simulink model "SAR_sw_neg"  (R2018b)
settings: Solver=VariableStepAuto  StartTime=0.0  StopTime=10.0  RelTol=1e-3
libraries: simulink_extras x11
settings Model: Creator=iamcy  LastModifiedBy=iamcy

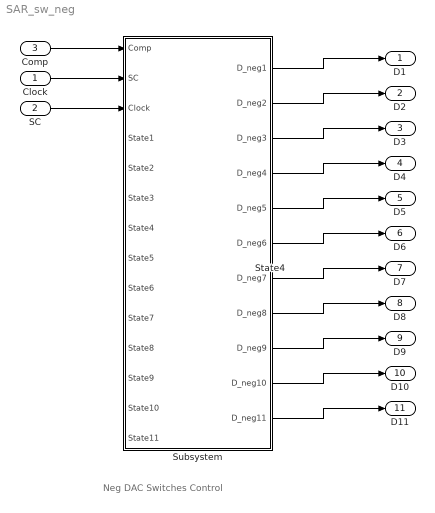
== system SAR_sw_neg ==
  note: Neg DAC Switches Control
  Clock : Inport
  SC : Inport  Port=2
  Comp : Inport  Port=3
  State4 : Inport  Port=4
  Subsystem : Subsystem
  D1 : Outport
  D2 : Outport  Port=2
  D3 : Outport  Port=3
  D4 : Outport  Port=4
  D5 : Outport  Port=5
  D6 : Outport  Port=6
  D7 : Outport  Port=7
  D8 : Outport  Port=8
  D9 : Outport  Port=9
  D10 : Outport  Port=10
  D11 : Outport  Port=11
  wires:
  Comp/1 -> Subsystem/1(Comp)
  Clock/1 -> Subsystem/2(SC)
  SC/1 -> Subsystem/3(Clock)
  Subsystem/1(D_neg1) -> D1/1
  Subsystem/2(D_neg2) -> D2/1
  Subsystem/3(D_neg3) -> D3/1
  Subsystem/4(D_neg4) -> D4/1
  Subsystem/5(D_neg5) -> D5/1
  Subsystem/6(D_neg6) -> D6/1
  Subsystem/7(D_neg7) -> D7/1
  Subsystem/8(D_neg8) -> D8/1
  Subsystem/9(D_neg9) -> D9/1
  Subsystem/10(D_neg10) -> D10/1
  Subsystem/11(D_neg11) -> D11/1

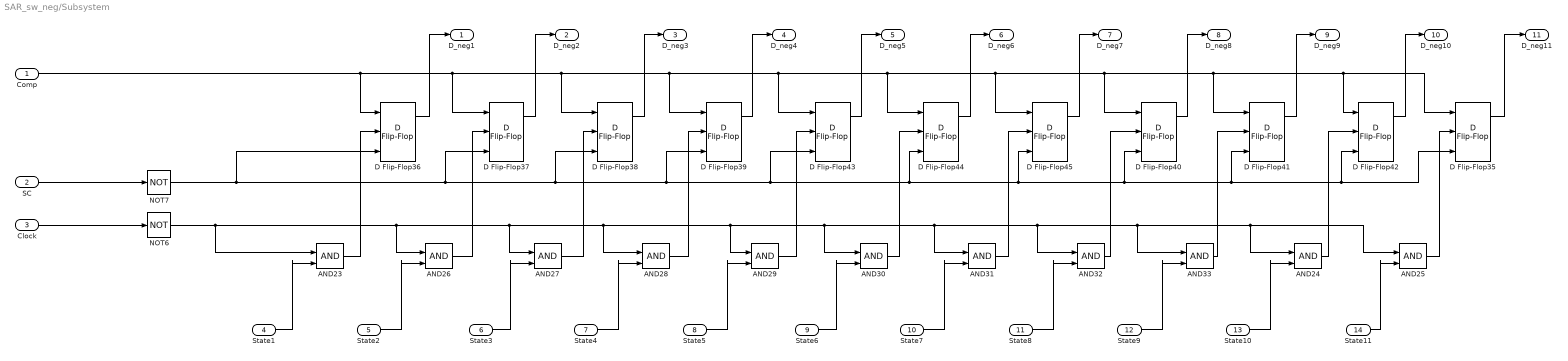
== system SAR_sw_neg/Subsystem ==
  Comp : Inport
  SC : Inport  Port=2
  Clock : Inport  Port=3
  State1 : Inport  Port=4
  State2 : Inport  Port=5
  State3 : Inport  Port=6
  State4 : Inport  Port=7
  State5 : Inport  Port=8
  State6 : Inport  Port=9
  State7 : Inport  Port=10
  State8 : Inport  Port=11
  State9 : Inport  Port=12
  State10 : Inport  Port=13
  State11 : Inport  Port=14
  AND{23..33} (11 alike) : Logic  IconShape=distinctive  AllPortsSameDT=off  OutDataTypeStr=boolean
  D Flip-Flop{35..45} (11 alike) : simulink_extras/Flip Flops/D Flip-Flop
      settings: SourceProductName=Simulink
  NOT6 : Logic  Operator=NOT  IconShape=distinctive  AllPortsSameDT=off  OutDataTypeStr=boolean
  NOT7 : Logic  Operator=NOT  IconShape=distinctive  AllPortsSameDT=off  OutDataTypeStr=boolean
  D_neg1 : Outport
  D_neg2 : Outport  Port=2
  D_neg3 : Outport  Port=3
  D_neg4 : Outport  Port=4
  D_neg5 : Outport  Port=5
  D_neg6 : Outport  Port=6
  D_neg7 : Outport  Port=7
  D_neg8 : Outport  Port=8
  D_neg9 : Outport  Port=9
  D_neg10 : Outport  Port=10
  D_neg11 : Outport  Port=11
  wires:
  NOT7/1 -> D Flip-Flop35/3, D Flip-Flop42/3, D Flip-Flop41/3, D Flip-Flop40/3, D Flip-Flop45/3, D Flip-Flop44/3, D Flip-Flop43/3, D Flip-Flop39/3, D Flip-Flop38/3, D Flip-Flop37/3, D Flip-Flop36/3
  D Flip-Flop41/1 -> D_neg9/1
  AND23/1 -> D Flip-Flop36/2
  State9/1 -> AND33/2
  Comp/1 -> D Flip-Flop35/1, D Flip-Flop42/1, D Flip-Flop41/1, D Flip-Flop40/1, D Flip-Flop45/1, D Flip-Flop44/1, D Flip-Flop43/1, D Flip-Flop39/1, D Flip-Flop38/1, D Flip-Flop37/1, D Flip-Flop36/1
  D Flip-Flop42/1 -> D_neg10/1
  AND27/1 -> D Flip-Flop38/2
  NOT6/1 -> AND25/1, AND24/1, AND33/1, AND32/1, AND31/1, AND30/1, AND29/1, AND28/1, AND27/1, AND26/1, AND23/1
  AND25/1 -> D Flip-Flop35/2
  AND29/1 -> D Flip-Flop43/2
  AND31/1 -> D Flip-Flop45/2
  AND28/1 -> D Flip-Flop39/2
  State1/1 -> AND23/2
  AND33/1 -> D Flip-Flop41/2
  D Flip-Flop45/1 -> D_neg7/1
  State5/1 -> AND29/2
  AND26/1 -> D Flip-Flop37/2
  AND24/1 -> D Flip-Flop42/2
  SC/1 -> NOT7/1
  AND32/1 -> D Flip-Flop40/2
  State10/1 -> AND24/2
  AND30/1 -> D Flip-Flop44/2
  D Flip-Flop38/1 -> D_neg3/1
  Clock/1 -> NOT6/1
  D Flip-Flop36/1 -> D_neg1/1
  D Flip-Flop37/1 -> D_neg2/1
  D Flip-Flop35/1 -> D_neg11/1
  D Flip-Flop43/1 -> D_neg5/1
  State4/1 -> AND28/2
  State3/1 -> AND27/2
  State2/1 -> AND26/2
  State8/1 -> AND32/2
  D Flip-Flop44/1 -> D_neg6/1
  State6/1 -> AND30/2
  State11/1 -> AND25/2
  D Flip-Flop40/1 -> D_neg8/1
  State7/1 -> AND31/2
  D Flip-Flop39/1 -> D_neg4/1
